simulink model "directcoupledPMDCmotorload"  (Simulink 7.7)
settings: Solver=ode45  StartTime=0.0  StopTime=100  RelTol=1e-3
libraries: elec_lib x72, fl_lib x14, nesl_utility x6
settings Model: Creator=Satellite  LastModifiedBy=Satellite

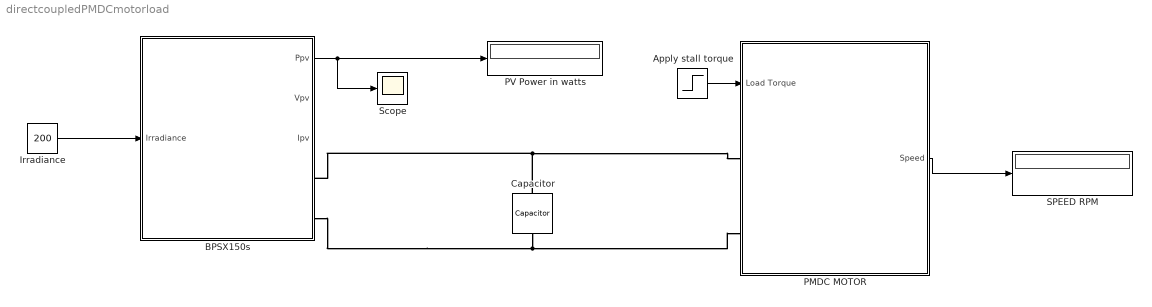
== system directcoupledPMDCmotorload ==
  " Irradiance" : Constant  Value=200
  Apply stall torque : Step  Time=0.001  After=-1.7  SampleTime=0
  BPSX150s : Subsystem
  Capacitor : fl_lib/Electrical/Electrical Elements/Capacitor  SystemSampleTime=-1  c=1e-6 F  v0=0 V  r=1e-6 Ohm  g=0 1/Ohm  i_Log=off  v_Log=off  vc_Log=off  LocalVarNames=|i|v|vc  LocalVarDescs=|i|v|Internal variable for voltage across capacitor term  LocalVarLogging=[0 0 0]
  PMDC MOTOR : Subsystem
  PV Power in watts : Display
  SPEED RPM : Display
  Scope : Scope
      settings: TimeRange=10  YMin=0  YMax=160
  wires:
  " Irradiance"/1 -> BPSX150s/1(Irradiance)
  BPSX150s/1(Ppv) -> PV Power in watts/1, Scope/1
  Apply stall torque/1 -> PMDC MOTOR/1(Load Torque)
  PMDC MOTOR/1(Speed) -> SPEED RPM/1
  connections:
  Capacitor/LConn1 -- BPSX150s/RConn1 -- PMDC MOTOR/LConn1
  BPSX150s/RConn2 -- PMDC MOTOR/LConn2 -- Capacitor/RConn1

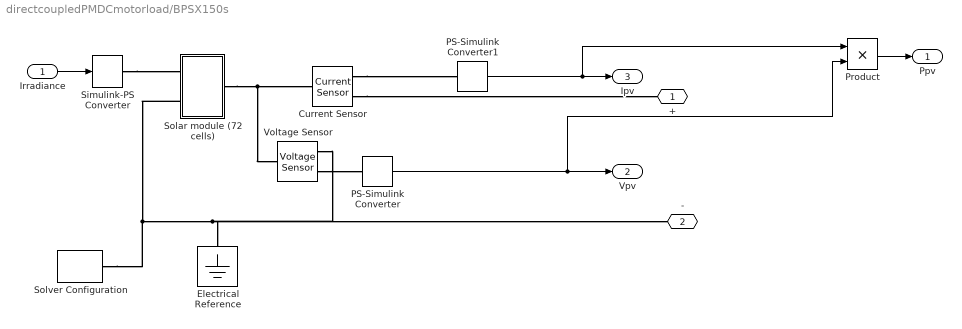
== system directcoupledPMDCmotorload/BPSX150s ==
  Irradiance : Inport
  Current Sensor : fl_lib/Electrical/Electrical Sensors/Current Sensor  SystemSampleTime=-1  i1_Log=off  v1_Log=off  LocalVarNames=|i1|v1  LocalVarDescs=|i1|v1  LocalVarLogging=[0 0]
  Electrical Reference : fl_lib/Electrical/Electrical Elements/Electrical Reference  SystemSampleTime=-1  i_Log=off  LocalVarNames=|i  LocalVarDescs=|i  LocalVarLogging=0
  PS-Simulink Converter : nesl_utility/PS-Simulink Converter  SystemSampleTime=-1  PhysicalDomain=network_engine_domain  LeftPortType=input  RightPortType=output  SubClassName=ps_output  Unit=1  AffineConversion=off
  PS-Simulink Converter1 : nesl_utility/PS-Simulink Converter  SystemSampleTime=-1  PhysicalDomain=network_engine_domain  LeftPortType=input  RightPortType=output  SubClassName=ps_output  Unit=1  AffineConversion=off
  Product : Product  RndMeth=Zero
  Simulink-PS Converter : nesl_utility/Simulink-PS Converter  SystemSampleTime=-1  PhysicalDomain=network_engine_domain  LeftPortType=input  RightPortType=output  SubClassName=ps_input  Unit=1  AffineConversion=off  InputFilterTimeConstant=.001  UdotUserProvided=0
  Solar module (72 cells) : Subsystem
  Solver Configuration : nesl_utility/Solver Configuration  SystemSampleTime=-1  PhysicalDomain=network_engine_domain  LeftPortType=input  RightPortType=generic  SubClassName=solver  Accelerate=off  Profile=off  ResidualTolerance=1e-9  MaxNonlinIter=3  MaxModeIter=2  DoFixedCost=on  UseLocalSampling=off  DoDC=off  LinearAlgebra=Sparse  LocalSolverSampleTime=.001  LocalSolverChoice=NE_BACKWARD_EULER_ADVANCER  UseLocalSolver=on
  Voltage Sensor : fl_lib/Electrical/Electrical Sensors/Voltage Sensor  SystemSampleTime=-1  i1_Log=off  v1_Log=off  LocalVarNames=|i1|v1  LocalVarDescs=|i1|v1  LocalVarLogging=[0 0]
  + : PMIOPort  Port=1  Side=Right
  - : PMIOPort  Port=2  Side=Right
  Ppv : Outport
  Vpv : Outport  Port=2
  Ipv : Outport  Port=3
  wires:
  Irradiance/1 -> Simulink-PS Converter/1
  PS-Simulink Converter1/1 -> Ipv/1, Product/1
  PS-Simulink Converter/1 -> Vpv/1, Product/2
  Product/1 -> Ppv/1
  connections:
  Simulink-PS Converter/RConn1 -- Solar module (72 cells)/LConn1
  Solar module (72 cells)/LConn2 -- Voltage Sensor/RConn2 -- -/RConn1 -- Electrical Reference/LConn1 -- Solver Configuration/RConn1
  Solar module (72 cells)/RConn1 -- Current Sensor/LConn1 -- Voltage Sensor/LConn1
  Current Sensor/RConn1 -- PS-Simulink Converter1/LConn1
  Voltage Sensor/RConn1 -- PS-Simulink Converter/LConn1
  Current Sensor/RConn2 -- +/RConn1

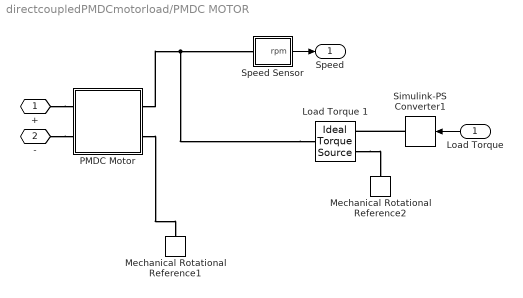
== system directcoupledPMDCmotorload/PMDC MOTOR ==
  Load Torque : Inport
  Load Torque 1 : fl_lib/Mechanical/Mechanical Sources/Ideal Torque Source  SystemSampleTime=-1  w_Log=off  t_Log=off  LocalVarNames=|torque|rel_velocity|power  LocalVarDescs=|Torque (N*m)|Relative velocity (rad/s)|Power generated by the source (W)  LocalVarLogging=[0 0 0]
  Mechanical Rotational Reference1 : fl_lib/Mechanical/Rotational Elements/Mechanical Rotational Reference  SystemSampleTime=-1  t_Log=off  LocalVarNames=|t  LocalVarDescs=|t  LocalVarLogging=[]
  Mechanical Rotational Reference2 : fl_lib/Mechanical/Rotational Elements/Mechanical Rotational Reference  SystemSampleTime=-1  t_Log=off  LocalVarNames=|t  LocalVarDescs=|t  LocalVarLogging=[]
  PMDC Motor : Subsystem
  Simulink-PS Converter1 : nesl_utility/Simulink-PS Converter  SystemSampleTime=-1  PhysicalDomain=network_engine_domain  LeftPortType=input  RightPortType=output  SubClassName=ps_input  Unit=1  AffineConversion=off  InputFilterTimeConstant=.001  UdotUserProvided=0
  Speed Sensor : Subsystem
  + : PMIOPort  Port=1  Side=Left
  - : PMIOPort  Port=2  Side=Left
  Speed : Outport
  wires:
  Speed Sensor/1(rpm) -> Speed/1
  Load Torque/1 -> Simulink-PS Converter1/1
  connections:
  Load Torque 1/LConn1 -- PMDC Motor/RConn1 -- Speed Sensor/LConn1
  Simulink-PS Converter1/RConn1 -- Load Torque 1/RConn1
  Load Torque 1/RConn2 -- Mechanical Rotational Reference2/LConn1
  PMDC Motor/RConn2 -- Mechanical Rotational Reference1/LConn1
  +/RConn1 -- PMDC Motor/LConn1
  -/RConn1 -- PMDC Motor/LConn2

== system directcoupledPMDCmotorload/BPSX150s/Solar module (72 cells) ==
  36 solarceel : Subsystem
  36 solarceel1 : Subsystem
  Ir : PMIOPort  Port=1  Side=Left
  + : PMIOPort  Port=2  Side=Right
  - : PMIOPort  Port=3  Side=Left
  connections:
  Ir/RConn1 -- 36 solarceel/LConn1 -- 36 solarceel1/LConn1
  36 solarceel/RConn1 -- 36 solarceel1/LConn2
  +/RConn1 -- 36 solarceel1/RConn1
  -/RConn1 -- 36 solarceel/LConn2

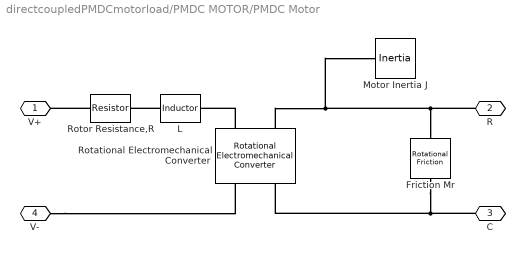
== system directcoupledPMDCmotorload/PMDC MOTOR/PMDC Motor ==
  Friction Mr : fl_lib/Mechanical/Rotational Elements/Rotational Friction  SystemSampleTime=-1  brkwy_trq=0.02e-3 N*m  Col_trq=0.02e-3 N*m  visc_coef=0.02 N*m/(rad/s)  trans_coef=10 s/rad  vel_thr=0.1 rad/s  t_Log=off  w_Log=off  LocalVarNames=|friction_torque|rel_velocity|power  LocalVarDescs=|Friction torque (N*m)|Relative velocity (rad/s)|Power (W)  LocalVarLogging=[0 0 0]
  L : fl_lib/Electrical/Electrical Elements/Inductor  SystemSampleTime=-1  l=10 mH  i0=0 A  r=0 Ohm  g=1e-09 1/Ohm  i_Log=off  v_Log=off  i_L_Log=off  LocalVarNames=|current|voltage|power  LocalVarDescs=|Inductor current (A) |Voltage across inductor (V)|Power (W)  LocalVarLogging=[0 0 0]
  Motor Inertia J : fl_lib/Mechanical/Rotational Elements/Inertia  SystemSampleTime=-1  inertia=0.05 kg*m^2  initial_velocity=0 rad/s  t_Log=off  LocalVarNames=|torque|velocity  LocalVarDescs=|Inertia torque (N*m)|Inertia absolute velocity (rad/s)  LocalVarLogging=[0 0]
  Rotational Electromechanical Converter : fl_lib/Electrical/Electrical Elements/Rotational Electromechanical Converter  SystemSampleTime=-1  K=1.8 V/(rad/s)  i_Log=off  v_Log=off  t_Log=off  w_Log=off  LocalVarNames=|current|voltage|power|torque|speed  LocalVarDescs=|Current (A)|Voltage (V)|Power (W)|Torque (Nm)|Angular speed (rad/s)  LocalVarLogging=[0 0 0 0 0]
  Rotor Resistance,R : fl_lib/Electrical/Electrical Elements/Resistor  Tag=Factory Generic  SystemSampleTime=-1  R=0.2 Ohm  i_Log=off  v_Log=off  LocalVarNames=|current|voltage|power  LocalVarDescs=|Resistor current (A)|Voltage across resistor (V)|Power (W)  LocalVarLogging=[0 0 0]
  V+ : PMIOPort  Port=1  Side=Left
  R : PMIOPort  Port=2  Side=Right
  C : PMIOPort  Port=3  Side=Right
  V- : PMIOPort  Port=4  Side=Left
  connections:
  Rotational Electromechanical Converter/LConn1 -- L/RConn1
  V-/RConn1 -- Rotational Electromechanical Converter/RConn1
  Rotor Resistance,R/LConn1 -- V+/RConn1
  L/LConn1 -- Rotor Resistance,R/RConn1
  R/RConn1 -- Rotational Electromechanical Converter/LConn2 -- Motor Inertia J/LConn1 -- Friction Mr/LConn1
  C/RConn1 -- Rotational Electromechanical Converter/RConn2 -- Friction Mr/RConn1

== system directcoupledPMDCmotorload/PMDC MOTOR/Speed Sensor ==
  Ideal Rotational Motion Sensor : fl_lib/Mechanical/Mechanical Sensors/Ideal Rotational Motion Sensor  SystemSampleTime=-1  offset=0 rad  w_Log=off  t_Log=off  phi_Log=off  LocalVarNames=|w|t|phi  LocalVarDescs=|w|t|phi  LocalVarLogging=[]
  Mechanical Rotational Reference : fl_lib/Mechanical/Rotational Elements/Mechanical Rotational Reference  SystemSampleTime=-1  t_Log=off  LocalVarNames=|t  LocalVarDescs=|t  LocalVarLogging=[]
  PS-Simulink Converter 2 : nesl_utility/PS-Simulink Converter  SystemSampleTime=-1  PhysicalDomain=network_engine_domain  LeftPortType=input  RightPortType=output  SubClassName=ps_output  Unit=rpm  AffineConversion=off
  R : PMIOPort  Port=1  Side=Left
  rpm : Outport
  wires:
  PS-Simulink Converter 2/1 -> rpm/1
  connections:
  R/RConn1 -- Ideal Rotational Motion Sensor/LConn1
  Ideal Rotational Motion Sensor/RConn1 -- Mechanical Rotational Reference/LConn1
  Ideal Rotational Motion Sensor/RConn2 -- PS-Simulink Converter 2/LConn1

== system directcoupledPMDCmotorload/BPSX150s/Solar module (72 cells)/36 solarceel ==
  18 solar cells : Subsystem
  18 solar cells1 : Subsystem
  Ir : PMIOPort  Port=1  Side=Left
  + : PMIOPort  Port=2  Side=Right
  - : PMIOPort  Port=3  Side=Left
  connections:
  Ir/RConn1 -- 18 solar cells1/LConn1 -- 18 solar cells/LConn1
  18 solar cells/RConn1 -- 18 solar cells1/LConn2
  +/RConn1 -- 18 solar cells1/RConn1
  -/RConn1 -- 18 solar cells/LConn2

== system directcoupledPMDCmotorload/BPSX150s/Solar module (72 cells)/36 solarceel1 ==
  18 solar cells : Subsystem
  18 solar cells1 : Subsystem
  Ir : PMIOPort  Port=1  Side=Left
  + : PMIOPort  Port=2  Side=Right
  - : PMIOPort  Port=3  Side=Left
  connections:
  18 solar cells/LConn1 -- Ir/RConn1 -- 18 solar cells1/LConn1
  18 solar cells/RConn1 -- 18 solar cells1/LConn2
  +/RConn1 -- 18 solar cells1/RConn1
  -/RConn1 -- 18 solar cells/LConn2

== system directcoupledPMDCmotorload/BPSX150s/Solar module (72 cells)/36 solarceel/18 solar cells ==
  6solarcells : Subsystem
  6solarcells1 : Subsystem
  6solarcells2 : Subsystem
  + : PMIOPort  Port=1  Side=Right
  Ir : PMIOPort  Port=2  Side=Left
  - : PMIOPort  Port=3  Side=Left
  connections:
  Ir/RConn1 -- 6solarcells1/LConn1 -- 6solarcells/LConn1 -- 6solarcells2/LConn1
  6solarcells/RConn1 -- 6solarcells1/LConn2
  6solarcells1/RConn1 -- 6solarcells2/LConn2
  +/RConn1 -- 6solarcells2/RConn1
  -/RConn1 -- 6solarcells/LConn2

== system directcoupledPMDCmotorload/BPSX150s/Solar module (72 cells)/36 solarceel/18 solar cells1 ==
  6solarcells : Subsystem
  6solarcells1 : Subsystem
  6solarcells2 : Subsystem
  + : PMIOPort  Port=1  Side=Right
  Ir : PMIOPort  Port=2  Side=Left
  - : PMIOPort  Port=3  Side=Left
  connections:
  6solarcells1/LConn1 -- 6solarcells/LConn1 -- Ir/RConn1 -- 6solarcells2/LConn1
  6solarcells/RConn1 -- 6solarcells1/LConn2
  6solarcells1/RConn1 -- 6solarcells2/LConn2
  +/RConn1 -- 6solarcells2/RConn1
  -/RConn1 -- 6solarcells/LConn2

== system directcoupledPMDCmotorload/BPSX150s/Solar module (72 cells)/36 solarceel1/18 solar cells ==
  6solarcells : Subsystem
  6solarcells1 : Subsystem
  6solarcells2 : Subsystem
  + : PMIOPort  Port=1  Side=Right
  Ir : PMIOPort  Port=2  Side=Left
  - : PMIOPort  Port=3  Side=Left
  connections:
  6solarcells1/LConn1 -- 6solarcells/LConn1 -- Ir/RConn1 -- 6solarcells2/LConn1
  6solarcells/RConn1 -- 6solarcells1/LConn2
  6solarcells1/RConn1 -- 6solarcells2/LConn2
  +/RConn1 -- 6solarcells2/RConn1
  -/RConn1 -- 6solarcells/LConn2

== system directcoupledPMDCmotorload/BPSX150s/Solar module (72 cells)/36 solarceel1/18 solar cells1 ==
  6solarcells : Subsystem
  6solarcells1 : Subsystem
  6solarcells2 : Subsystem
  + : PMIOPort  Port=1  Side=Right
  Ir : PMIOPort  Port=2  Side=Left
  - : PMIOPort  Port=3  Side=Left
  connections:
  6solarcells1/LConn1 -- 6solarcells/LConn1 -- Ir/RConn1 -- 6solarcells2/LConn1
  6solarcells/RConn1 -- 6solarcells1/LConn2
  6solarcells1/RConn1 -- 6solarcells2/LConn2
  +/RConn1 -- 6solarcells2/RConn1
  -/RConn1 -- 6solarcells/LConn2

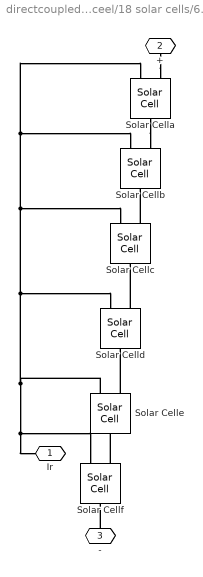
== system directcoupledPMDCmotorload/BPSX150s/Solar module (72 cells)/36 solarceel/18 solar cells/6solarcells ==
  Solar Cella : elec_lib/Sources/Solar Cell  SystemSampleTime=-1  prm=1  Isc=4.75 A  Voc=0.6 V  Is=1e-6 A  Is2=0 A  Iph=7.34 A  Ir0=1000 W/m^2  ec=1.6  N2=2  Rs=5.1e-3 Ohm  Rp=Inf Ohm  TIPH1=0.65e-3 1/K  EG=1.12 eV  TXIS1=3  TXIS2=3  TRS1=0  TRP1=0  TFIXED=25 C  Tmeas=25 C  LocalVarLogging=[]
  Solar Cellb : elec_lib/Sources/Solar Cell  SystemSampleTime=-1  prm=1  Isc=4.75 A  Voc=0.6 V  Is=1e-6 A  Is2=0 A  Iph=7.34 A  Ir0=1000 W/m^2  ec=1.6  N2=2  Rs=5.1e-3 Ohm  Rp=Inf Ohm  TIPH1=0.65e-3 1/K  EG=1.12 eV  TXIS1=3  TXIS2=3  TRS1=0  TRP1=0  TFIXED=25 C  Tmeas=25 C  LocalVarLogging=[]
  Solar Cellc : elec_lib/Sources/Solar Cell  SystemSampleTime=-1  prm=1  Isc=4.75 A  Voc=0.6 V  Is=1e-6 A  Is2=0 A  Iph=7.34 A  Ir0=1000 W/m^2  ec=1.6  N2=2  Rs=5.1e-3 Ohm  Rp=Inf Ohm  TIPH1=0.65e-3 1/K  EG=1.12 eV  TXIS1=3  TXIS2=3  TRS1=0  TRP1=0  TFIXED=25 C  Tmeas=25 C  LocalVarLogging=[]
  Solar Celld : elec_lib/Sources/Solar Cell  SystemSampleTime=-1  prm=1  Isc=4.75 A  Voc=0.6 V  Is=1e-6 A  Is2=0 A  Iph=7.34 A  Ir0=1000 W/m^2  ec=1.6  N2=2  Rs=5.1e-3 Ohm  Rp=Inf Ohm  TIPH1=0.65e-3 1/K  EG=1.12 eV  TXIS1=3  TXIS2=3  TRS1=0  TRP1=0  TFIXED=25 C  Tmeas=25 C  LocalVarLogging=[]
  Solar Celle : elec_lib/Sources/Solar Cell  SystemSampleTime=-1  prm=1  Isc=4.75 A  Voc=0.6 V  Is=1e-6 A  Is2=0 A  Iph=7.34 A  Ir0=1000 W/m^2  ec=1.6  N2=2  Rs=5.1e-3 Ohm  Rp=Inf Ohm  TIPH1=0.65e-3 1/K  EG=1.12 eV  TXIS1=3  TXIS2=3  TRS1=0  TRP1=0  TFIXED=25 C  Tmeas=25 C  LocalVarLogging=[]
  Solar Cellf : elec_lib/Sources/Solar Cell  SystemSampleTime=-1  prm=1  Isc=4.75 A  Voc=0.6 V  Is=1e-6 A  Is2=0 A  Iph=7.34 A  Ir0=1000 W/m^2  ec=1.6  N2=2  Rs=5.1e-3 Ohm  Rp=Inf Ohm  TIPH1=0.65e-3 1/K  EG=1.12 eV  TXIS1=3  TXIS2=3  TRS1=0  TRP1=0  TFIXED=25 C  Tmeas=25 C  LocalVarLogging=[]
  Ir : PMIOPort  Port=1  Side=Left
  + : PMIOPort  Port=2  Side=Right
  - : PMIOPort  Port=3  Side=Left
  connections:
  Ir/RConn1 -- Solar Celle/LConn1 -- Solar Celld/LConn1 -- Solar Cellc/LConn1 -- Solar Cellb/LConn1 -- Solar Cella/LConn1 -- Solar Cellf/LConn1
  Solar Cella/RConn1 -- Solar Cellb/LConn2
  Solar Cellc/LConn2 -- Solar Cellb/RConn1
  Solar Celld/LConn2 -- Solar Cellc/RConn1
  Solar Celle/LConn2 -- Solar Celld/RConn1
  Solar Cellf/LConn2 -- Solar Celle/RConn1
  +/RConn1 -- Solar Cella/LConn2
  -/RConn1 -- Solar Cellf/RConn1

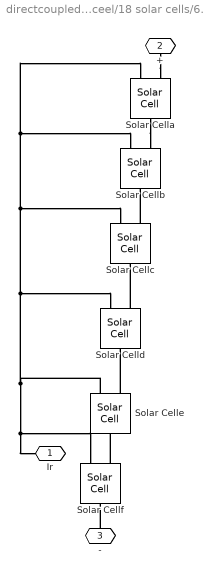
== system directcoupledPMDCmotorload/BPSX150s/Solar module (72 cells)/36 solarceel/18 solar cells/6solarcells1 ==
  Solar Cella : elec_lib/Sources/Solar Cell  SystemSampleTime=-1  prm=1  Isc=4.75 A  Voc=0.6 V  Is=1e-6 A  Is2=0 A  Iph=7.34 A  Ir0=1000 W/m^2  ec=1.6  N2=2  Rs=5.1e-3 Ohm  Rp=Inf Ohm  TIPH1=0.65e-3 1/K  EG=1.12 eV  TXIS1=3  TXIS2=3  TRS1=0  TRP1=0  TFIXED=25 C  Tmeas=25 C  LocalVarLogging=[]
  Solar Cellb : elec_lib/Sources/Solar Cell  SystemSampleTime=-1  prm=1  Isc=4.75 A  Voc=0.6 V  Is=1e-6 A  Is2=0 A  Iph=7.34 A  Ir0=1000 W/m^2  ec=1.6  N2=2  Rs=5.1e-3 Ohm  Rp=Inf Ohm  TIPH1=0.65e-3 1/K  EG=1.12 eV  TXIS1=3  TXIS2=3  TRS1=0  TRP1=0  TFIXED=25 C  Tmeas=25 C  LocalVarLogging=[]
  Solar Cellc : elec_lib/Sources/Solar Cell  SystemSampleTime=-1  prm=1  Isc=4.75 A  Voc=0.6 V  Is=1e-6 A  Is2=0 A  Iph=7.34 A  Ir0=1000 W/m^2  ec=1.6  N2=2  Rs=5.1e-3 Ohm  Rp=Inf Ohm  TIPH1=0.65e-3 1/K  EG=1.12 eV  TXIS1=3  TXIS2=3  TRS1=0  TRP1=0  TFIXED=25 C  Tmeas=25 C  LocalVarLogging=[]
  Solar Celld : elec_lib/Sources/Solar Cell  SystemSampleTime=-1  prm=1  Isc=4.75 A  Voc=0.6 V  Is=1e-6 A  Is2=0 A  Iph=7.34 A  Ir0=1000 W/m^2  ec=1.6  N2=2  Rs=5.1e-3 Ohm  Rp=Inf Ohm  TIPH1=0.65e-3 1/K  EG=1.12 eV  TXIS1=3  TXIS2=3  TRS1=0  TRP1=0  TFIXED=25 C  Tmeas=25 C  LocalVarLogging=[]
  Solar Celle : elec_lib/Sources/Solar Cell  SystemSampleTime=-1  prm=1  Isc=4.75 A  Voc=0.6 V  Is=1e-6 A  Is2=0 A  Iph=7.34 A  Ir0=1000 W/m^2  ec=1.6  N2=2  Rs=5.1e-3 Ohm  Rp=Inf Ohm  TIPH1=0.65e-3 1/K  EG=1.12 eV  TXIS1=3  TXIS2=3  TRS1=0  TRP1=0  TFIXED=25 C  Tmeas=25 C  LocalVarLogging=[]
  Solar Cellf : elec_lib/Sources/Solar Cell  SystemSampleTime=-1  prm=1  Isc=4.75 A  Voc=0.6 V  Is=1e-6 A  Is2=0 A  Iph=7.34 A  Ir0=1000 W/m^2  ec=1.6  N2=2  Rs=5.1e-3 Ohm  Rp=Inf Ohm  TIPH1=0.65e-3 1/K  EG=1.12 eV  TXIS1=3  TXIS2=3  TRS1=0  TRP1=0  TFIXED=25 C  Tmeas=25 C  LocalVarLogging=[]
  Ir : PMIOPort  Port=1  Side=Left
  + : PMIOPort  Port=2  Side=Right
  - : PMIOPort  Port=3  Side=Left
  connections:
  Solar Celle/LConn1 -- Solar Cellf/LConn1 -- Ir/RConn1 -- Solar Celld/LConn1 -- Solar Cellc/LConn1 -- Solar Cella/LConn1 -- Solar Cellb/LConn1
  Solar Cella/RConn1 -- Solar Cellb/LConn2
  Solar Cellc/LConn2 -- Solar Cellb/RConn1
  Solar Celld/LConn2 -- Solar Cellc/RConn1
  Solar Celle/LConn2 -- Solar Celld/RConn1
  Solar Cellf/LConn2 -- Solar Celle/RConn1
  +/RConn1 -- Solar Cella/LConn2
  -/RConn1 -- Solar Cellf/RConn1

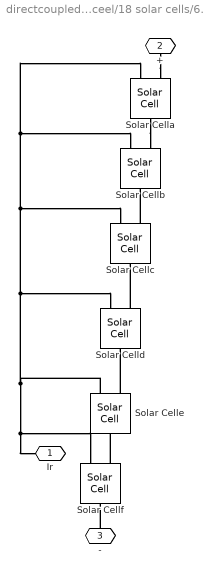
== system directcoupledPMDCmotorload/BPSX150s/Solar module (72 cells)/36 solarceel/18 solar cells/6solarcells2 ==
  Solar Cella : elec_lib/Sources/Solar Cell  SystemSampleTime=-1  prm=1  Isc=4.75 A  Voc=0.6 V  Is=1e-6 A  Is2=0 A  Iph=7.34 A  Ir0=1000 W/m^2  ec=1.6  N2=2  Rs=5.1e-3 Ohm  Rp=Inf Ohm  TIPH1=0.65e-3 1/K  EG=1.12 eV  TXIS1=3  TXIS2=3  TRS1=0  TRP1=0  TFIXED=25 C  Tmeas=25 C  LocalVarLogging=[]
  Solar Cellb : elec_lib/Sources/Solar Cell  SystemSampleTime=-1  prm=1  Isc=4.75 A  Voc=0.6 V  Is=1e-6 A  Is2=0 A  Iph=7.34 A  Ir0=1000 W/m^2  ec=1.6  N2=2  Rs=5.1e-3 Ohm  Rp=Inf Ohm  TIPH1=0.65e-3 1/K  EG=1.12 eV  TXIS1=3  TXIS2=3  TRS1=0  TRP1=0  TFIXED=25 C  Tmeas=25 C  LocalVarLogging=[]
  Solar Cellc : elec_lib/Sources/Solar Cell  SystemSampleTime=-1  prm=1  Isc=4.75 A  Voc=0.6 V  Is=1e-6 A  Is2=0 A  Iph=7.34 A  Ir0=1000 W/m^2  ec=1.6  N2=2  Rs=5.1e-3 Ohm  Rp=Inf Ohm  TIPH1=0.65e-3 1/K  EG=1.12 eV  TXIS1=3  TXIS2=3  TRS1=0  TRP1=0  TFIXED=25 C  Tmeas=25 C  LocalVarLogging=[]
  Solar Celld : elec_lib/Sources/Solar Cell  SystemSampleTime=-1  prm=1  Isc=4.75 A  Voc=0.6 V  Is=1e-6 A  Is2=0 A  Iph=7.34 A  Ir0=1000 W/m^2  ec=1.6  N2=2  Rs=5.1e-3 Ohm  Rp=Inf Ohm  TIPH1=0.65e-3 1/K  EG=1.12 eV  TXIS1=3  TXIS2=3  TRS1=0  TRP1=0  TFIXED=25 C  Tmeas=25 C  LocalVarLogging=[]
  Solar Celle : elec_lib/Sources/Solar Cell  SystemSampleTime=-1  prm=1  Isc=4.75 A  Voc=0.6 V  Is=1e-6 A  Is2=0 A  Iph=7.34 A  Ir0=1000 W/m^2  ec=1.6  N2=2  Rs=5.1e-3 Ohm  Rp=Inf Ohm  TIPH1=0.65e-3 1/K  EG=1.12 eV  TXIS1=3  TXIS2=3  TRS1=0  TRP1=0  TFIXED=25 C  Tmeas=25 C  LocalVarLogging=[]
  Solar Cellf : elec_lib/Sources/Solar Cell  SystemSampleTime=-1  prm=1  Isc=4.75 A  Voc=0.6 V  Is=1e-6 A  Is2=0 A  Iph=7.34 A  Ir0=1000 W/m^2  ec=1.6  N2=2  Rs=5.1e-3 Ohm  Rp=Inf Ohm  TIPH1=0.65e-3 1/K  EG=1.12 eV  TXIS1=3  TXIS2=3  TRS1=0  TRP1=0  TFIXED=25 C  Tmeas=25 C  LocalVarLogging=[]
  Ir : PMIOPort  Port=1  Side=Left
  + : PMIOPort  Port=2  Side=Right
  - : PMIOPort  Port=3  Side=Left
  connections:
  Solar Celle/LConn1 -- Solar Cellf/LConn1 -- Ir/RConn1 -- Solar Celld/LConn1 -- Solar Cellc/LConn1 -- Solar Cella/LConn1 -- Solar Cellb/LConn1
  Solar Cella/RConn1 -- Solar Cellb/LConn2
  Solar Cellc/LConn2 -- Solar Cellb/RConn1
  Solar Celld/LConn2 -- Solar Cellc/RConn1
  Solar Celle/LConn2 -- Solar Celld/RConn1
  Solar Cellf/LConn2 -- Solar Celle/RConn1
  +/RConn1 -- Solar Cella/LConn2
  -/RConn1 -- Solar Cellf/RConn1

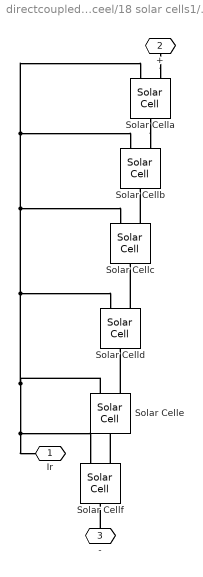
== system directcoupledPMDCmotorload/BPSX150s/Solar module (72 cells)/36 solarceel/18 solar cells1/6solarcells ==
  Solar Cella : elec_lib/Sources/Solar Cell  SystemSampleTime=-1  prm=1  Isc=4.75 A  Voc=0.6 V  Is=1e-6 A  Is2=0 A  Iph=7.34 A  Ir0=1000 W/m^2  ec=1.6  N2=2  Rs=5.1e-3 Ohm  Rp=Inf Ohm  TIPH1=0.65e-3 1/K  EG=1.12 eV  TXIS1=3  TXIS2=3  TRS1=0  TRP1=0  TFIXED=25 C  Tmeas=25 C  LocalVarLogging=[]
  Solar Cellb : elec_lib/Sources/Solar Cell  SystemSampleTime=-1  prm=1  Isc=4.75 A  Voc=0.6 V  Is=1e-6 A  Is2=0 A  Iph=7.34 A  Ir0=1000 W/m^2  ec=1.6  N2=2  Rs=5.1e-3 Ohm  Rp=Inf Ohm  TIPH1=0.65e-3 1/K  EG=1.12 eV  TXIS1=3  TXIS2=3  TRS1=0  TRP1=0  TFIXED=25 C  Tmeas=25 C  LocalVarLogging=[]
  Solar Cellc : elec_lib/Sources/Solar Cell  SystemSampleTime=-1  prm=1  Isc=4.75 A  Voc=0.6 V  Is=1e-6 A  Is2=0 A  Iph=7.34 A  Ir0=1000 W/m^2  ec=1.6  N2=2  Rs=5.1e-3 Ohm  Rp=Inf Ohm  TIPH1=0.65e-3 1/K  EG=1.12 eV  TXIS1=3  TXIS2=3  TRS1=0  TRP1=0  TFIXED=25 C  Tmeas=25 C  LocalVarLogging=[]
  Solar Celld : elec_lib/Sources/Solar Cell  SystemSampleTime=-1  prm=1  Isc=4.75 A  Voc=0.6 V  Is=1e-6 A  Is2=0 A  Iph=7.34 A  Ir0=1000 W/m^2  ec=1.6  N2=2  Rs=5.1e-3 Ohm  Rp=Inf Ohm  TIPH1=0.65e-3 1/K  EG=1.12 eV  TXIS1=3  TXIS2=3  TRS1=0  TRP1=0  TFIXED=25 C  Tmeas=25 C  LocalVarLogging=[]
  Solar Celle : elec_lib/Sources/Solar Cell  SystemSampleTime=-1  prm=1  Isc=4.75 A  Voc=0.6 V  Is=1e-6 A  Is2=0 A  Iph=7.34 A  Ir0=1000 W/m^2  ec=1.6  N2=2  Rs=5.1e-3 Ohm  Rp=Inf Ohm  TIPH1=0.65e-3 1/K  EG=1.12 eV  TXIS1=3  TXIS2=3  TRS1=0  TRP1=0  TFIXED=25 C  Tmeas=25 C  LocalVarLogging=[]
  Solar Cellf : elec_lib/Sources/Solar Cell  SystemSampleTime=-1  prm=1  Isc=4.75 A  Voc=0.6 V  Is=1e-6 A  Is2=0 A  Iph=7.34 A  Ir0=1000 W/m^2  ec=1.6  N2=2  Rs=5.1e-3 Ohm  Rp=Inf Ohm  TIPH1=0.65e-3 1/K  EG=1.12 eV  TXIS1=3  TXIS2=3  TRS1=0  TRP1=0  TFIXED=25 C  Tmeas=25 C  LocalVarLogging=[]
  Ir : PMIOPort  Port=1  Side=Left
  + : PMIOPort  Port=2  Side=Right
  - : PMIOPort  Port=3  Side=Left
  connections:
  Solar Celle/LConn1 -- Solar Cellf/LConn1 -- Ir/RConn1 -- Solar Celld/LConn1 -- Solar Cellc/LConn1 -- Solar Cella/LConn1 -- Solar Cellb/LConn1
  Solar Cella/RConn1 -- Solar Cellb/LConn2
  Solar Cellc/LConn2 -- Solar Cellb/RConn1
  Solar Celld/LConn2 -- Solar Cellc/RConn1
  Solar Celle/LConn2 -- Solar Celld/RConn1
  Solar Cellf/LConn2 -- Solar Celle/RConn1
  +/RConn1 -- Solar Cella/LConn2
  -/RConn1 -- Solar Cellf/RConn1

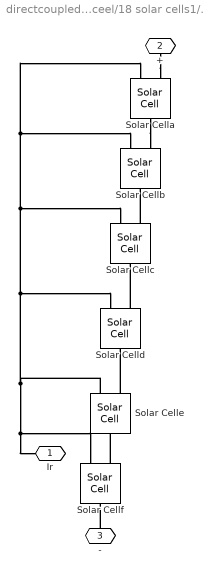
== system directcoupledPMDCmotorload/BPSX150s/Solar module (72 cells)/36 solarceel/18 solar cells1/6solarcells1 ==
  Solar Cella : elec_lib/Sources/Solar Cell  SystemSampleTime=-1  prm=1  Isc=4.75 A  Voc=0.6 V  Is=1e-6 A  Is2=0 A  Iph=7.34 A  Ir0=1000 W/m^2  ec=1.6  N2=2  Rs=5.1e-3 Ohm  Rp=Inf Ohm  TIPH1=0.65e-3 1/K  EG=1.12 eV  TXIS1=3  TXIS2=3  TRS1=0  TRP1=0  TFIXED=25 C  Tmeas=25 C  LocalVarLogging=[]
  Solar Cellb : elec_lib/Sources/Solar Cell  SystemSampleTime=-1  prm=1  Isc=4.75 A  Voc=0.6 V  Is=1e-6 A  Is2=0 A  Iph=7.34 A  Ir0=1000 W/m^2  ec=1.6  N2=2  Rs=5.1e-3 Ohm  Rp=Inf Ohm  TIPH1=0.65e-3 1/K  EG=1.12 eV  TXIS1=3  TXIS2=3  TRS1=0  TRP1=0  TFIXED=25 C  Tmeas=25 C  LocalVarLogging=[]
  Solar Cellc : elec_lib/Sources/Solar Cell  SystemSampleTime=-1  prm=1  Isc=4.75 A  Voc=0.6 V  Is=1e-6 A  Is2=0 A  Iph=7.34 A  Ir0=1000 W/m^2  ec=1.6  N2=2  Rs=5.1e-3 Ohm  Rp=Inf Ohm  TIPH1=0.65e-3 1/K  EG=1.12 eV  TXIS1=3  TXIS2=3  TRS1=0  TRP1=0  TFIXED=25 C  Tmeas=25 C  LocalVarLogging=[]
  Solar Celld : elec_lib/Sources/Solar Cell  SystemSampleTime=-1  prm=1  Isc=4.75 A  Voc=0.6 V  Is=1e-6 A  Is2=0 A  Iph=7.34 A  Ir0=1000 W/m^2  ec=1.6  N2=2  Rs=5.1e-3 Ohm  Rp=Inf Ohm  TIPH1=0.65e-3 1/K  EG=1.12 eV  TXIS1=3  TXIS2=3  TRS1=0  TRP1=0  TFIXED=25 C  Tmeas=25 C  LocalVarLogging=[]
  Solar Celle : elec_lib/Sources/Solar Cell  SystemSampleTime=-1  prm=1  Isc=4.75 A  Voc=0.6 V  Is=1e-6 A  Is2=0 A  Iph=7.34 A  Ir0=1000 W/m^2  ec=1.6  N2=2  Rs=5.1e-3 Ohm  Rp=Inf Ohm  TIPH1=0.65e-3 1/K  EG=1.12 eV  TXIS1=3  TXIS2=3  TRS1=0  TRP1=0  TFIXED=25 C  Tmeas=25 C  LocalVarLogging=[]
  Solar Cellf : elec_lib/Sources/Solar Cell  SystemSampleTime=-1  prm=1  Isc=4.75 A  Voc=0.6 V  Is=1e-6 A  Is2=0 A  Iph=7.34 A  Ir0=1000 W/m^2  ec=1.6  N2=2  Rs=5.1e-3 Ohm  Rp=Inf Ohm  TIPH1=0.65e-3 1/K  EG=1.12 eV  TXIS1=3  TXIS2=3  TRS1=0  TRP1=0  TFIXED=25 C  Tmeas=25 C  LocalVarLogging=[]
  Ir : PMIOPort  Port=1  Side=Left
  + : PMIOPort  Port=2  Side=Right
  - : PMIOPort  Port=3  Side=Left
  connections:
  Solar Celle/LConn1 -- Solar Cellf/LConn1 -- Ir/RConn1 -- Solar Celld/LConn1 -- Solar Cellc/LConn1 -- Solar Cella/LConn1 -- Solar Cellb/LConn1
  Solar Cella/RConn1 -- Solar Cellb/LConn2
  Solar Cellc/LConn2 -- Solar Cellb/RConn1
  Solar Celld/LConn2 -- Solar Cellc/RConn1
  Solar Celle/LConn2 -- Solar Celld/RConn1
  Solar Cellf/LConn2 -- Solar Celle/RConn1
  +/RConn1 -- Solar Cella/LConn2
  -/RConn1 -- Solar Cellf/RConn1

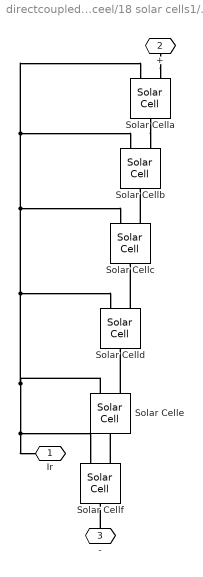
== system directcoupledPMDCmotorload/BPSX150s/Solar module (72 cells)/36 solarceel/18 solar cells1/6solarcells2 ==
  Solar Cella : elec_lib/Sources/Solar Cell  SystemSampleTime=-1  prm=1  Isc=4.75 A  Voc=0.6 V  Is=1e-6 A  Is2=0 A  Iph=7.34 A  Ir0=1000 W/m^2  ec=1.6  N2=2  Rs=5.1e-3 Ohm  Rp=Inf Ohm  TIPH1=0.65e-3 1/K  EG=1.12 eV  TXIS1=3  TXIS2=3  TRS1=0  TRP1=0  TFIXED=25 C  Tmeas=25 C  LocalVarLogging=[]
  Solar Cellb : elec_lib/Sources/Solar Cell  SystemSampleTime=-1  prm=1  Isc=4.75 A  Voc=0.6 V  Is=1e-6 A  Is2=0 A  Iph=7.34 A  Ir0=1000 W/m^2  ec=1.6  N2=2  Rs=5.1e-3 Ohm  Rp=Inf Ohm  TIPH1=0.65e-3 1/K  EG=1.12 eV  TXIS1=3  TXIS2=3  TRS1=0  TRP1=0  TFIXED=25 C  Tmeas=25 C  LocalVarLogging=[]
  Solar Cellc : elec_lib/Sources/Solar Cell  SystemSampleTime=-1  prm=1  Isc=4.75 A  Voc=0.6 V  Is=1e-6 A  Is2=0 A  Iph=7.34 A  Ir0=1000 W/m^2  ec=1.6  N2=2  Rs=5.1e-3 Ohm  Rp=Inf Ohm  TIPH1=0.65e-3 1/K  EG=1.12 eV  TXIS1=3  TXIS2=3  TRS1=0  TRP1=0  TFIXED=25 C  Tmeas=25 C  LocalVarLogging=[]
  Solar Celld : elec_lib/Sources/Solar Cell  SystemSampleTime=-1  prm=1  Isc=4.75 A  Voc=0.6 V  Is=1e-6 A  Is2=0 A  Iph=7.34 A  Ir0=1000 W/m^2  ec=1.6  N2=2  Rs=5.1e-3 Ohm  Rp=Inf Ohm  TIPH1=0.65e-3 1/K  EG=1.12 eV  TXIS1=3  TXIS2=3  TRS1=0  TRP1=0  TFIXED=25 C  Tmeas=25 C  LocalVarLogging=[]
  Solar Celle : elec_lib/Sources/Solar Cell  SystemSampleTime=-1  prm=1  Isc=4.75 A  Voc=0.6 V  Is=1e-6 A  Is2=0 A  Iph=7.34 A  Ir0=1000 W/m^2  ec=1.6  N2=2  Rs=5.1e-3 Ohm  Rp=Inf Ohm  TIPH1=0.65e-3 1/K  EG=1.12 eV  TXIS1=3  TXIS2=3  TRS1=0  TRP1=0  TFIXED=25 C  Tmeas=25 C  LocalVarLogging=[]
  Solar Cellf : elec_lib/Sources/Solar Cell  SystemSampleTime=-1  prm=1  Isc=4.75 A  Voc=0.6 V  Is=1e-6 A  Is2=0 A  Iph=7.34 A  Ir0=1000 W/m^2  ec=1.6  N2=2  Rs=5.1e-3 Ohm  Rp=Inf Ohm  TIPH1=0.65e-3 1/K  EG=1.12 eV  TXIS1=3  TXIS2=3  TRS1=0  TRP1=0  TFIXED=25 C  Tmeas=25 C  LocalVarLogging=[]
  Ir : PMIOPort  Port=1  Side=Left
  + : PMIOPort  Port=2  Side=Right
  - : PMIOPort  Port=3  Side=Left
  connections:
  Solar Celle/LConn1 -- Solar Cellf/LConn1 -- Ir/RConn1 -- Solar Celld/LConn1 -- Solar Cellc/LConn1 -- Solar Cella/LConn1 -- Solar Cellb/LConn1
  Solar Cella/RConn1 -- Solar Cellb/LConn2
  Solar Cellc/LConn2 -- Solar Cellb/RConn1
  Solar Celld/LConn2 -- Solar Cellc/RConn1
  Solar Celle/LConn2 -- Solar Celld/RConn1
  Solar Cellf/LConn2 -- Solar Celle/RConn1
  +/RConn1 -- Solar Cella/LConn2
  -/RConn1 -- Solar Cellf/RConn1

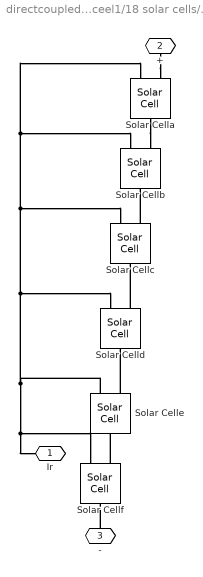
== system directcoupledPMDCmotorload/BPSX150s/Solar module (72 cells)/36 solarceel1/18 solar cells/6solarcells ==
  Solar Cella : elec_lib/Sources/Solar Cell  SystemSampleTime=-1  prm=1  Isc=4.75 A  Voc=0.6 V  Is=1e-6 A  Is2=0 A  Iph=7.34 A  Ir0=1000 W/m^2  ec=1.6  N2=2  Rs=5.1e-3 Ohm  Rp=Inf Ohm  TIPH1=0.65e-3 1/K  EG=1.12 eV  TXIS1=3  TXIS2=3  TRS1=0  TRP1=0  TFIXED=25 C  Tmeas=25 C  LocalVarLogging=[]
  Solar Cellb : elec_lib/Sources/Solar Cell  SystemSampleTime=-1  prm=1  Isc=4.75 A  Voc=0.6 V  Is=1e-6 A  Is2=0 A  Iph=7.34 A  Ir0=1000 W/m^2  ec=1.6  N2=2  Rs=5.1e-3 Ohm  Rp=Inf Ohm  TIPH1=0.65e-3 1/K  EG=1.12 eV  TXIS1=3  TXIS2=3  TRS1=0  TRP1=0  TFIXED=25 C  Tmeas=25 C  LocalVarLogging=[]
  Solar Cellc : elec_lib/Sources/Solar Cell  SystemSampleTime=-1  prm=1  Isc=4.75 A  Voc=0.6 V  Is=1e-6 A  Is2=0 A  Iph=7.34 A  Ir0=1000 W/m^2  ec=1.6  N2=2  Rs=5.1e-3 Ohm  Rp=Inf Ohm  TIPH1=0.65e-3 1/K  EG=1.12 eV  TXIS1=3  TXIS2=3  TRS1=0  TRP1=0  TFIXED=25 C  Tmeas=25 C  LocalVarLogging=[]
  Solar Celld : elec_lib/Sources/Solar Cell  SystemSampleTime=-1  prm=1  Isc=4.75 A  Voc=0.6 V  Is=1e-6 A  Is2=0 A  Iph=7.34 A  Ir0=1000 W/m^2  ec=1.6  N2=2  Rs=5.1e-3 Ohm  Rp=Inf Ohm  TIPH1=0.65e-3 1/K  EG=1.12 eV  TXIS1=3  TXIS2=3  TRS1=0  TRP1=0  TFIXED=25 C  Tmeas=25 C  LocalVarLogging=[]
  Solar Celle : elec_lib/Sources/Solar Cell  SystemSampleTime=-1  prm=1  Isc=4.75 A  Voc=0.6 V  Is=1e-6 A  Is2=0 A  Iph=7.34 A  Ir0=1000 W/m^2  ec=1.6  N2=2  Rs=5.1e-3 Ohm  Rp=Inf Ohm  TIPH1=0.65e-3 1/K  EG=1.12 eV  TXIS1=3  TXIS2=3  TRS1=0  TRP1=0  TFIXED=25 C  Tmeas=25 C  LocalVarLogging=[]
  Solar Cellf : elec_lib/Sources/Solar Cell  SystemSampleTime=-1  prm=1  Isc=4.75 A  Voc=0.6 V  Is=1e-6 A  Is2=0 A  Iph=7.34 A  Ir0=1000 W/m^2  ec=1.6  N2=2  Rs=5.1e-3 Ohm  Rp=Inf Ohm  TIPH1=0.65e-3 1/K  EG=1.12 eV  TXIS1=3  TXIS2=3  TRS1=0  TRP1=0  TFIXED=25 C  Tmeas=25 C  LocalVarLogging=[]
  Ir : PMIOPort  Port=1  Side=Left
  + : PMIOPort  Port=2  Side=Right
  - : PMIOPort  Port=3  Side=Left
  connections:
  Solar Celle/LConn1 -- Solar Cellf/LConn1 -- Ir/RConn1 -- Solar Celld/LConn1 -- Solar Cellc/LConn1 -- Solar Cella/LConn1 -- Solar Cellb/LConn1
  Solar Cella/RConn1 -- Solar Cellb/LConn2
  Solar Cellc/LConn2 -- Solar Cellb/RConn1
  Solar Celld/LConn2 -- Solar Cellc/RConn1
  Solar Celle/LConn2 -- Solar Celld/RConn1
  Solar Cellf/LConn2 -- Solar Celle/RConn1
  +/RConn1 -- Solar Cella/LConn2
  -/RConn1 -- Solar Cellf/RConn1

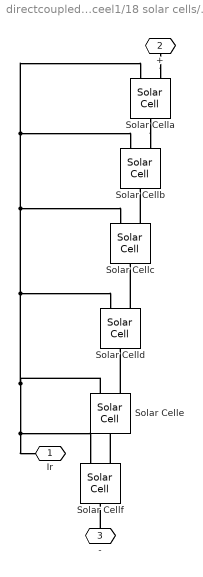
== system directcoupledPMDCmotorload/BPSX150s/Solar module (72 cells)/36 solarceel1/18 solar cells/6solarcells1 ==
  Solar Cella : elec_lib/Sources/Solar Cell  SystemSampleTime=-1  prm=1  Isc=4.75 A  Voc=0.6 V  Is=1e-6 A  Is2=0 A  Iph=7.34 A  Ir0=1000 W/m^2  ec=1.6  N2=2  Rs=5.1e-3 Ohm  Rp=Inf Ohm  TIPH1=0.65e-3 1/K  EG=1.12 eV  TXIS1=3  TXIS2=3  TRS1=0  TRP1=0  TFIXED=25 C  Tmeas=25 C  LocalVarLogging=[]
  Solar Cellb : elec_lib/Sources/Solar Cell  SystemSampleTime=-1  prm=1  Isc=4.75 A  Voc=0.6 V  Is=1e-6 A  Is2=0 A  Iph=7.34 A  Ir0=1000 W/m^2  ec=1.6  N2=2  Rs=5.1e-3 Ohm  Rp=Inf Ohm  TIPH1=0.65e-3 1/K  EG=1.12 eV  TXIS1=3  TXIS2=3  TRS1=0  TRP1=0  TFIXED=25 C  Tmeas=25 C  LocalVarLogging=[]
  Solar Cellc : elec_lib/Sources/Solar Cell  SystemSampleTime=-1  prm=1  Isc=4.75 A  Voc=0.6 V  Is=1e-6 A  Is2=0 A  Iph=7.34 A  Ir0=1000 W/m^2  ec=1.6  N2=2  Rs=5.1e-3 Ohm  Rp=Inf Ohm  TIPH1=0.65e-3 1/K  EG=1.12 eV  TXIS1=3  TXIS2=3  TRS1=0  TRP1=0  TFIXED=25 C  Tmeas=25 C  LocalVarLogging=[]
  Solar Celld : elec_lib/Sources/Solar Cell  SystemSampleTime=-1  prm=1  Isc=4.75 A  Voc=0.6 V  Is=1e-6 A  Is2=0 A  Iph=7.34 A  Ir0=1000 W/m^2  ec=1.6  N2=2  Rs=5.1e-3 Ohm  Rp=Inf Ohm  TIPH1=0.65e-3 1/K  EG=1.12 eV  TXIS1=3  TXIS2=3  TRS1=0  TRP1=0  TFIXED=25 C  Tmeas=25 C  LocalVarLogging=[]
  Solar Celle : elec_lib/Sources/Solar Cell  SystemSampleTime=-1  prm=1  Isc=4.75 A  Voc=0.6 V  Is=1e-6 A  Is2=0 A  Iph=7.34 A  Ir0=1000 W/m^2  ec=1.6  N2=2  Rs=5.1e-3 Ohm  Rp=Inf Ohm  TIPH1=0.65e-3 1/K  EG=1.12 eV  TXIS1=3  TXIS2=3  TRS1=0  TRP1=0  TFIXED=25 C  Tmeas=25 C  LocalVarLogging=[]
  Solar Cellf : elec_lib/Sources/Solar Cell  SystemSampleTime=-1  prm=1  Isc=4.75 A  Voc=0.6 V  Is=1e-6 A  Is2=0 A  Iph=7.34 A  Ir0=1000 W/m^2  ec=1.6  N2=2  Rs=5.1e-3 Ohm  Rp=Inf Ohm  TIPH1=0.65e-3 1/K  EG=1.12 eV  TXIS1=3  TXIS2=3  TRS1=0  TRP1=0  TFIXED=25 C  Tmeas=25 C  LocalVarLogging=[]
  Ir : PMIOPort  Port=1  Side=Left
  + : PMIOPort  Port=2  Side=Right
  - : PMIOPort  Port=3  Side=Left
  connections:
  Solar Celle/LConn1 -- Solar Cellf/LConn1 -- Ir/RConn1 -- Solar Celld/LConn1 -- Solar Cellc/LConn1 -- Solar Cella/LConn1 -- Solar Cellb/LConn1
  Solar Cella/RConn1 -- Solar Cellb/LConn2
  Solar Cellc/LConn2 -- Solar Cellb/RConn1
  Solar Celld/LConn2 -- Solar Cellc/RConn1
  Solar Celle/LConn2 -- Solar Celld/RConn1
  Solar Cellf/LConn2 -- Solar Celle/RConn1
  +/RConn1 -- Solar Cella/LConn2
  -/RConn1 -- Solar Cellf/RConn1

== system directcoupledPMDCmotorload/BPSX150s/Solar module (72 cells)/36 solarceel1/18 solar cells/6solarcells2 ==
  Solar Cella : elec_lib/Sources/Solar Cell  SystemSampleTime=-1  prm=1  Isc=4.75 A  Voc=0.6 V  Is=1e-6 A  Is2=0 A  Iph=7.34 A  Ir0=1000 W/m^2  ec=1.6  N2=2  Rs=5.1e-3 Ohm  Rp=Inf Ohm  TIPH1=0.65e-3 1/K  EG=1.12 eV  TXIS1=3  TXIS2=3  TRS1=0  TRP1=0  TFIXED=25 C  Tmeas=25 C  LocalVarLogging=[]
  Solar Cellb : elec_lib/Sources/Solar Cell  SystemSampleTime=-1  prm=1  Isc=4.75 A  Voc=0.6 V  Is=1e-6 A  Is2=0 A  Iph=7.34 A  Ir0=1000 W/m^2  ec=1.6  N2=2  Rs=5.1e-3 Ohm  Rp=Inf Ohm  TIPH1=0.65e-3 1/K  EG=1.12 eV  TXIS1=3  TXIS2=3  TRS1=0  TRP1=0  TFIXED=25 C  Tmeas=25 C  LocalVarLogging=[]
  Solar Cellc : elec_lib/Sources/Solar Cell  SystemSampleTime=-1  prm=1  Isc=4.75 A  Voc=0.6 V  Is=1e-6 A  Is2=0 A  Iph=7.34 A  Ir0=1000 W/m^2  ec=1.6  N2=2  Rs=5.1e-3 Ohm  Rp=Inf Ohm  TIPH1=0.65e-3 1/K  EG=1.12 eV  TXIS1=3  TXIS2=3  TRS1=0  TRP1=0  TFIXED=25 C  Tmeas=25 C  LocalVarLogging=[]
  Solar Celld : elec_lib/Sources/Solar Cell  SystemSampleTime=-1  prm=1  Isc=4.75 A  Voc=0.6 V  Is=1e-6 A  Is2=0 A  Iph=7.34 A  Ir0=1000 W/m^2  ec=1.6  N2=2  Rs=5.1e-3 Ohm  Rp=Inf Ohm  TIPH1=0.65e-3 1/K  EG=1.12 eV  TXIS1=3  TXIS2=3  TRS1=0  TRP1=0  TFIXED=25 C  Tmeas=25 C  LocalVarLogging=[]
  Solar Celle : elec_lib/Sources/Solar Cell  SystemSampleTime=-1  prm=1  Isc=4.75 A  Voc=0.6 V  Is=1e-6 A  Is2=0 A  Iph=7.34 A  Ir0=1000 W/m^2  ec=1.6  N2=2  Rs=5.1e-3 Ohm  Rp=Inf Ohm  TIPH1=0.65e-3 1/K  EG=1.12 eV  TXIS1=3  TXIS2=3  TRS1=0  TRP1=0  TFIXED=25 C  Tmeas=25 C  LocalVarLogging=[]
  Solar Cellf : elec_lib/Sources/Solar Cell  SystemSampleTime=-1  prm=1  Isc=4.75 A  Voc=0.6 V  Is=1e-6 A  Is2=0 A  Iph=7.34 A  Ir0=1000 W/m^2  ec=1.6  N2=2  Rs=5.1e-3 Ohm  Rp=Inf Ohm  TIPH1=0.65e-3 1/K  EG=1.12 eV  TXIS1=3  TXIS2=3  TRS1=0  TRP1=0  TFIXED=25 C  Tmeas=25 C  LocalVarLogging=[]
  Ir : PMIOPort  Port=1  Side=Left
  + : PMIOPort  Port=2  Side=Right
  - : PMIOPort  Port=3  Side=Left
  connections:
  Solar Celle/LConn1 -- Solar Cellf/LConn1 -- Ir/RConn1 -- Solar Celld/LConn1 -- Solar Cellc/LConn1 -- Solar Cella/LConn1 -- Solar Cellb/LConn1
  Solar Cella/RConn1 -- Solar Cellb/LConn2
  Solar Cellc/LConn2 -- Solar Cellb/RConn1
  Solar Celld/LConn2 -- Solar Cellc/RConn1
  Solar Celle/LConn2 -- Solar Celld/RConn1
  Solar Cellf/LConn2 -- Solar Celle/RConn1
  +/RConn1 -- Solar Cella/LConn2
  -/RConn1 -- Solar Cellf/RConn1

== system directcoupledPMDCmotorload/BPSX150s/Solar module (72 cells)/36 solarceel1/18 solar cells1/6solarcells ==
  Solar Cella : elec_lib/Sources/Solar Cell  SystemSampleTime=-1  prm=1  Isc=4.75 A  Voc=0.6 V  Is=1e-6 A  Is2=0 A  Iph=7.34 A  Ir0=1000 W/m^2  ec=1.6  N2=2  Rs=5.1e-3 Ohm  Rp=Inf Ohm  TIPH1=0.65e-3 1/K  EG=1.12 eV  TXIS1=3  TXIS2=3  TRS1=0  TRP1=0  TFIXED=25 C  Tmeas=25 C  LocalVarLogging=[]
  Solar Cellb : elec_lib/Sources/Solar Cell  SystemSampleTime=-1  prm=1  Isc=4.75 A  Voc=0.6 V  Is=1e-6 A  Is2=0 A  Iph=7.34 A  Ir0=1000 W/m^2  ec=1.6  N2=2  Rs=5.1e-3 Ohm  Rp=Inf Ohm  TIPH1=0.65e-3 1/K  EG=1.12 eV  TXIS1=3  TXIS2=3  TRS1=0  TRP1=0  TFIXED=25 C  Tmeas=25 C  LocalVarLogging=[]
  Solar Cellc : elec_lib/Sources/Solar Cell  SystemSampleTime=-1  prm=1  Isc=4.75 A  Voc=0.6 V  Is=1e-6 A  Is2=0 A  Iph=7.34 A  Ir0=1000 W/m^2  ec=1.6  N2=2  Rs=5.1e-3 Ohm  Rp=Inf Ohm  TIPH1=0.65e-3 1/K  EG=1.12 eV  TXIS1=3  TXIS2=3  TRS1=0  TRP1=0  TFIXED=25 C  Tmeas=25 C  LocalVarLogging=[]
  Solar Celld : elec_lib/Sources/Solar Cell  SystemSampleTime=-1  prm=1  Isc=4.75 A  Voc=0.6 V  Is=1e-6 A  Is2=0 A  Iph=7.34 A  Ir0=1000 W/m^2  ec=1.6  N2=2  Rs=5.1e-3 Ohm  Rp=Inf Ohm  TIPH1=0.65e-3 1/K  EG=1.12 eV  TXIS1=3  TXIS2=3  TRS1=0  TRP1=0  TFIXED=25 C  Tmeas=25 C  LocalVarLogging=[]
  Solar Celle : elec_lib/Sources/Solar Cell  SystemSampleTime=-1  prm=1  Isc=4.75 A  Voc=0.6 V  Is=1e-6 A  Is2=0 A  Iph=7.34 A  Ir0=1000 W/m^2  ec=1.6  N2=2  Rs=5.1e-3 Ohm  Rp=Inf Ohm  TIPH1=0.65e-3 1/K  EG=1.12 eV  TXIS1=3  TXIS2=3  TRS1=0  TRP1=0  TFIXED=25 C  Tmeas=25 C  LocalVarLogging=[]
  Solar Cellf : elec_lib/Sources/Solar Cell  SystemSampleTime=-1  prm=1  Isc=4.75 A  Voc=0.6 V  Is=1e-6 A  Is2=0 A  Iph=7.34 A  Ir0=1000 W/m^2  ec=1.6  N2=2  Rs=5.1e-3 Ohm  Rp=Inf Ohm  TIPH1=0.65e-3 1/K  EG=1.12 eV  TXIS1=3  TXIS2=3  TRS1=0  TRP1=0  TFIXED=25 C  Tmeas=25 C  LocalVarLogging=[]
  Ir : PMIOPort  Port=1  Side=Left
  + : PMIOPort  Port=2  Side=Right
  - : PMIOPort  Port=3  Side=Left
  connections:
  Solar Celle/LConn1 -- Solar Cellf/LConn1 -- Ir/RConn1 -- Solar Celld/LConn1 -- Solar Cellc/LConn1 -- Solar Cella/LConn1 -- Solar Cellb/LConn1
  Solar Cella/RConn1 -- Solar Cellb/LConn2
  Solar Cellc/LConn2 -- Solar Cellb/RConn1
  Solar Celld/LConn2 -- Solar Cellc/RConn1
  Solar Celle/LConn2 -- Solar Celld/RConn1
  Solar Cellf/LConn2 -- Solar Celle/RConn1
  +/RConn1 -- Solar Cella/LConn2
  -/RConn1 -- Solar Cellf/RConn1

== system directcoupledPMDCmotorload/BPSX150s/Solar module (72 cells)/36 solarceel1/18 solar cells1/6solarcells1 ==
  Solar Cella : elec_lib/Sources/Solar Cell  SystemSampleTime=-1  prm=1  Isc=4.75 A  Voc=0.6 V  Is=1e-6 A  Is2=0 A  Iph=7.34 A  Ir0=1000 W/m^2  ec=1.6  N2=2  Rs=5.1e-3 Ohm  Rp=Inf Ohm  TIPH1=0.65e-3 1/K  EG=1.12 eV  TXIS1=3  TXIS2=3  TRS1=0  TRP1=0  TFIXED=25 C  Tmeas=25 C  LocalVarLogging=[]
  Solar Cellb : elec_lib/Sources/Solar Cell  SystemSampleTime=-1  prm=1  Isc=4.75 A  Voc=0.6 V  Is=1e-6 A  Is2=0 A  Iph=7.34 A  Ir0=1000 W/m^2  ec=1.6  N2=2  Rs=5.1e-3 Ohm  Rp=Inf Ohm  TIPH1=0.65e-3 1/K  EG=1.12 eV  TXIS1=3  TXIS2=3  TRS1=0  TRP1=0  TFIXED=25 C  Tmeas=25 C  LocalVarLogging=[]
  Solar Cellc : elec_lib/Sources/Solar Cell  SystemSampleTime=-1  prm=1  Isc=4.75 A  Voc=0.6 V  Is=1e-6 A  Is2=0 A  Iph=7.34 A  Ir0=1000 W/m^2  ec=1.6  N2=2  Rs=5.1e-3 Ohm  Rp=Inf Ohm  TIPH1=0.65e-3 1/K  EG=1.12 eV  TXIS1=3  TXIS2=3  TRS1=0  TRP1=0  TFIXED=25 C  Tmeas=25 C  LocalVarLogging=[]
  Solar Celld : elec_lib/Sources/Solar Cell  SystemSampleTime=-1  prm=1  Isc=4.75 A  Voc=0.6 V  Is=1e-6 A  Is2=0 A  Iph=7.34 A  Ir0=1000 W/m^2  ec=1.6  N2=2  Rs=5.1e-3 Ohm  Rp=Inf Ohm  TIPH1=0.65e-3 1/K  EG=1.12 eV  TXIS1=3  TXIS2=3  TRS1=0  TRP1=0  TFIXED=25 C  Tmeas=25 C  LocalVarLogging=[]
  Solar Celle : elec_lib/Sources/Solar Cell  SystemSampleTime=-1  prm=1  Isc=4.75 A  Voc=0.6 V  Is=1e-6 A  Is2=0 A  Iph=7.34 A  Ir0=1000 W/m^2  ec=1.6  N2=2  Rs=5.1e-3 Ohm  Rp=Inf Ohm  TIPH1=0.65e-3 1/K  EG=1.12 eV  TXIS1=3  TXIS2=3  TRS1=0  TRP1=0  TFIXED=25 C  Tmeas=25 C  LocalVarLogging=[]
  Solar Cellf : elec_lib/Sources/Solar Cell  SystemSampleTime=-1  prm=1  Isc=4.75 A  Voc=0.6 V  Is=1e-6 A  Is2=0 A  Iph=7.34 A  Ir0=1000 W/m^2  ec=1.6  N2=2  Rs=5.1e-3 Ohm  Rp=Inf Ohm  TIPH1=0.65e-3 1/K  EG=1.12 eV  TXIS1=3  TXIS2=3  TRS1=0  TRP1=0  TFIXED=25 C  Tmeas=25 C  LocalVarLogging=[]
  Ir : PMIOPort  Port=1  Side=Left
  + : PMIOPort  Port=2  Side=Right
  - : PMIOPort  Port=3  Side=Left
  connections:
  Solar Celle/LConn1 -- Solar Cellf/LConn1 -- Ir/RConn1 -- Solar Celld/LConn1 -- Solar Cellc/LConn1 -- Solar Cella/LConn1 -- Solar Cellb/LConn1
  Solar Cella/RConn1 -- Solar Cellb/LConn2
  Solar Cellc/LConn2 -- Solar Cellb/RConn1
  Solar Celld/LConn2 -- Solar Cellc/RConn1
  Solar Celle/LConn2 -- Solar Celld/RConn1
  Solar Cellf/LConn2 -- Solar Celle/RConn1
  +/RConn1 -- Solar Cella/LConn2
  -/RConn1 -- Solar Cellf/RConn1

== system directcoupledPMDCmotorload/BPSX150s/Solar module (72 cells)/36 solarceel1/18 solar cells1/6solarcells2 ==
  Solar Cella : elec_lib/Sources/Solar Cell  SystemSampleTime=-1  prm=1  Isc=4.75 A  Voc=0.6 V  Is=1e-6 A  Is2=0 A  Iph=7.34 A  Ir0=1000 W/m^2  ec=1.6  N2=2  Rs=5.1e-3 Ohm  Rp=Inf Ohm  TIPH1=0.65e-3 1/K  EG=1.12 eV  TXIS1=3  TXIS2=3  TRS1=0  TRP1=0  TFIXED=25 C  Tmeas=25 C  LocalVarLogging=[]
  Solar Cellb : elec_lib/Sources/Solar Cell  SystemSampleTime=-1  prm=1  Isc=4.75 A  Voc=0.6 V  Is=1e-6 A  Is2=0 A  Iph=7.34 A  Ir0=1000 W/m^2  ec=1.6  N2=2  Rs=5.1e-3 Ohm  Rp=Inf Ohm  TIPH1=0.65e-3 1/K  EG=1.12 eV  TXIS1=3  TXIS2=3  TRS1=0  TRP1=0  TFIXED=25 C  Tmeas=25 C  LocalVarLogging=[]
  Solar Cellc : elec_lib/Sources/Solar Cell  SystemSampleTime=-1  prm=1  Isc=4.75 A  Voc=0.6 V  Is=1e-6 A  Is2=0 A  Iph=7.34 A  Ir0=1000 W/m^2  ec=1.6  N2=2  Rs=5.1e-3 Ohm  Rp=Inf Ohm  TIPH1=0.65e-3 1/K  EG=1.12 eV  TXIS1=3  TXIS2=3  TRS1=0  TRP1=0  TFIXED=25 C  Tmeas=25 C  LocalVarLogging=[]
  Solar Celld : elec_lib/Sources/Solar Cell  SystemSampleTime=-1  prm=1  Isc=4.75 A  Voc=0.6 V  Is=1e-6 A  Is2=0 A  Iph=7.34 A  Ir0=1000 W/m^2  ec=1.6  N2=2  Rs=5.1e-3 Ohm  Rp=Inf Ohm  TIPH1=0.65e-3 1/K  EG=1.12 eV  TXIS1=3  TXIS2=3  TRS1=0  TRP1=0  TFIXED=25 C  Tmeas=25 C  LocalVarLogging=[]
  Solar Celle : elec_lib/Sources/Solar Cell  SystemSampleTime=-1  prm=1  Isc=4.75 A  Voc=0.6 V  Is=1e-6 A  Is2=0 A  Iph=7.34 A  Ir0=1000 W/m^2  ec=1.6  N2=2  Rs=5.1e-3 Ohm  Rp=Inf Ohm  TIPH1=0.65e-3 1/K  EG=1.12 eV  TXIS1=3  TXIS2=3  TRS1=0  TRP1=0  TFIXED=25 C  Tmeas=25 C  LocalVarLogging=[]
  Solar Cellf : elec_lib/Sources/Solar Cell  SystemSampleTime=-1  prm=1  Isc=4.75 A  Voc=0.6 V  Is=1e-6 A  Is2=0 A  Iph=7.34 A  Ir0=1000 W/m^2  ec=1.6  N2=2  Rs=5.1e-3 Ohm  Rp=Inf Ohm  TIPH1=0.65e-3 1/K  EG=1.12 eV  TXIS1=3  TXIS2=3  TRS1=0  TRP1=0  TFIXED=25 C  Tmeas=25 C  LocalVarLogging=[]
  Ir : PMIOPort  Port=1  Side=Left
  + : PMIOPort  Port=2  Side=Right
  - : PMIOPort  Port=3  Side=Left
  connections:
  Solar Celle/LConn1 -- Solar Cellf/LConn1 -- Ir/RConn1 -- Solar Celld/LConn1 -- Solar Cellc/LConn1 -- Solar Cella/LConn1 -- Solar Cellb/LConn1
  Solar Cella/RConn1 -- Solar Cellb/LConn2
  Solar Cellc/LConn2 -- Solar Cellb/RConn1
  Solar Celld/LConn2 -- Solar Cellc/RConn1
  Solar Celle/LConn2 -- Solar Celld/RConn1
  Solar Cellf/LConn2 -- Solar Celle/RConn1
  +/RConn1 -- Solar Cella/LConn2
  -/RConn1 -- Solar Cellf/RConn1
